simulink model "ukf_simple_model"  (R2014b)
settings: Solver=FixedStepAuto  StartTime=0.0  StopTime=tdur  FixedStep=dt  RelTol=1e-3
values from neighbouring files (symbols this model uses):
  dt = 0.05    [ukf_simple_run.m]
  sig_noise = 1e-2    (= 0.01)    [ukf_simple_run.m]
  u_0 = [0;0;0]    [ukf_simple_run.m]
  x_0 = [deg2rad(15);0;5]    [ukf_simple_run.m]
settings Model: Creator=Rusty Goh  LastModifiedBy=root
settings DataIOCC: LimitDataPoints=off  SaveFormat=Dataset  SaveOutput=off
settings OptimizationCC: UseDivisionForNetSlopeComputation=off  LifeSpan=auto  SimCompilerOptimization=off
settings DebuggingCC: SolverPrmCheckMsg=none  FcnCallInpInsideContextMsg=error  FrameProcessingCompatibilityMsg=error  SFUnexpectedBacktrackingDiag=error  SFNoUnconditionalDefaultTransitionDiag=error
settings HardwareCC: ProdBitPerPointer=64  ProdLargestAtomicFloat=Float  ProdIntDivRoundTo=Zero  ProdEndianess=LittleEndian  ProdWordSize=64  ProdHWDeviceType=Intel->x86-64 (Windows64)
settings ModelReferenceCC: PropagateSignalLabelsOutOfModel=on
settings RTWCC: RTWCompilerOptimization=off
settings GRTTargetCC: TargetLangStandard=C99 (ISO)  GeneratePreprocessorConditionals=Use local settings

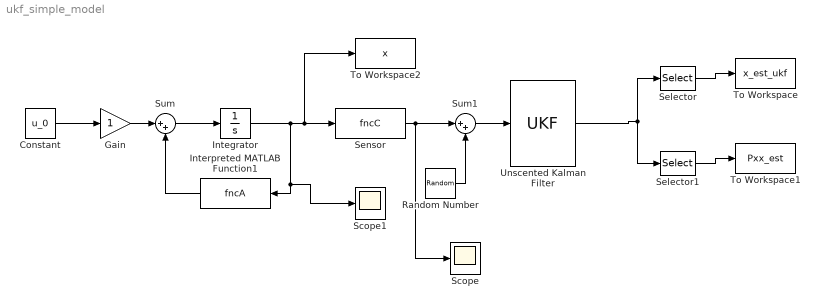
== system ukf_simple_model ==
  Constant : Constant  Value=u_0
  Gain : Gain
  Integrator : Integrator  InitialCondition=x_0
  Interpreted MATLAB Function1 : MATLABFcn  MATLABFcn=fncA  OutputDimensions=[3,1]  Output1D=off
  Random Number : RandomNumber  Variance=sig_noise^2  SampleTime=dt
  Scope : Scope
      settings: YMin=-0.04369  YMax=0.48598
  Scope1 : Scope
      settings: YMin=-0.213  YMax=0.2061
  Selector : Selector  NumberOfDimensions=2  InputPortWidth=3  IndexOptions=Index vector (dialog),Index vector (dialog)  Indices=[1:3],1  OutputSizes=1,1
  Selector1 : Selector  NumberOfDimensions=2  InputPortWidth=3  IndexOptions=Index vector (dialog),Index vector (dialog)  Indices=[1:3],[2:4]  OutputSizes=1,1
  "Sensor " : MATLABFcn  MATLABFcn=fncC  OutputDimensions=[1,1]  Output1D=off
  Sum : Sum  Inputs=|++
  Sum1 : Sum  Inputs=|++
  To Workspace : ToWorkspace  VariableName=x_est_ukf  SampleTime=dt
  To Workspace1 : ToWorkspace  VariableName=Pxx_est  SampleTime=dt
  To Workspace2 : ToWorkspace  VariableName=x  SampleTime=dt
  Unscented Kalman Filter : MATLABFcn  MATLABFcn=UKF  OutputDimensions=[3,4]  Output1D=off  SampleTime=dt
  wires:
  "Sensor "/1 -> Sum1/1, Scope/1
  Interpreted MATLAB Function1/1 -> Sum/2
  Sum/1 -> Integrator/1
  Gain/1 -> Sum/1
  Constant/1 -> Gain/1
  Unscented Kalman Filter/1 -> Selector1/1, Selector/1
  Selector/1 -> To Workspace/1
  Selector1/1 -> To Workspace1/1
  Integrator/1 -> Scope1/1, Interpreted MATLAB Function1/1, To Workspace2/1, "Sensor "/1
  Sum1/1 -> Unscented Kalman Filter/1
  Random Number/1 -> Sum1/2
